simulink model "planar_vtol_sim_HW_08"  (R2018a)
settings: Solver=ode45  StartTime=0.0  StopTime=100  MaxStep=1  MinStep=0.005  RelTol=1e-3
InitFcn:
  | planar_vtol_param
undefined symbols (not defined in the file or in its folder): Pa, planar_vtol_animation, planar_vtol_ctrl
settings Model: Creator=canla  LastModifiedBy=canla
settings OptimizationCC: LifeSpan=inf

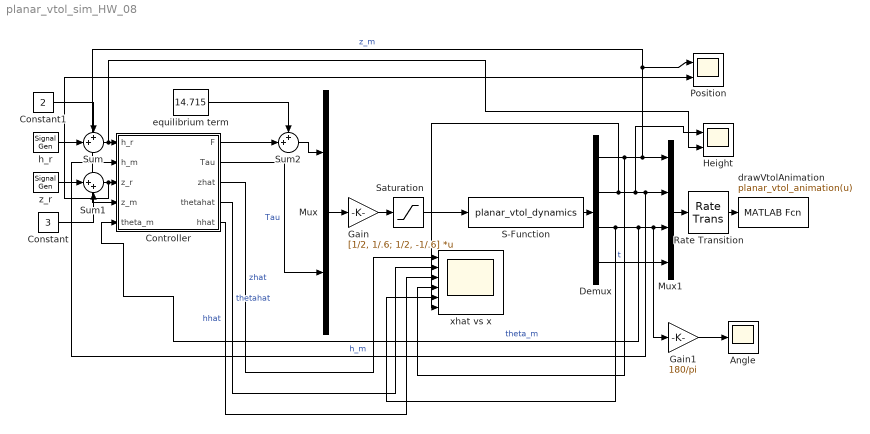
== system planar_vtol_sim_HW_08 ==
  Angle : Scope
  Constant : Constant  Value=3
  Constant1 : Constant  Value=2
  Controller : Subsystem
  Demux : Demux
  Gain : Gain  Gain=[1/2, 1/.6; 1/2, -1/.6]  Multiplication=Matrix(K*u)
  Gain1 : Gain  Gain=180/pi
  Height : Scope  NumInputPorts=2
  Mux : Mux  Inputs=2
  Mux1 : Mux
  Position : Scope  NumInputPorts=2
  Rate Transition : RateTransition  OutPortSampleTime=Pa.t_plot
  S-Function : S-Function  FunctionName=planar_vtol_dynamics  Parameters=Pa  SFunctionDeploymentMode=off  EnableBusSupport=off
  Saturation : Saturate  UpperLimit=Pa.F_max  LowerLimit=-Pa.F_max
  Sum : Sum  Inputs=++|
  Sum1 : Sum  Inputs=|++
  Sum2 : Sum  Inputs=++|
  drawVtolAnimation : MATLABFcn  MATLABFcn=planar_vtol_animation(u)  OutputDimensions=0
  equilibrium term : Constant  Value=14.715
  h_r : SignalGenerator  WaveForm=square  Amplitude=0.15  Frequency=0.03
  xhat vs x : Scope  NumInputPorts=6
  z_r : SignalGenerator  WaveForm=square  Amplitude=0.15  Frequency=0.03
  wires:
  Mux/1 -> Gain/1
  S-Function/1 -> Demux/1
  Demux/1 -> xhat vs x/4, Position/1, Controller/4(z_m), Mux1/1  "z_m"
  Demux/2 -> xhat vs x/6, Height/1, Controller/2(h_m), Mux1/2  "h_m"
  Demux/3 -> xhat vs x/5, Controller/5(theta_m), Gain1/1, Mux1/3  "theta_m"
  Demux/4 -> Mux1/4  "t"
  Mux1/1 -> Rate Transition/1
  Rate Transition/1 -> drawVtolAnimation/1
  Gain/1 -> Saturation/1
  Sum/1 -> Height/2, Controller/1(h_r)
  Sum1/1 -> Position/2, Controller/3(z_r)
  h_r/1 -> Sum/2
  z_r/1 -> Sum1/1
  Constant/1 -> Sum1/2
  Constant1/1 -> Sum/1
  Gain1/1 -> Angle/1
  Sum2/1 -> Mux/1
  Saturation/1 -> S-Function/1
  equilibrium term/1 -> Sum2/1
  Controller/1(F) -> Sum2/2
  Controller/3(zhat) -> xhat vs x/1  "zhat"
  Controller/4(thetahat) -> xhat vs x/2  "thetahat"
  Controller/5(hhat) -> xhat vs x/3  "hhat"
  Controller/2(Tau) -> Mux/2  "Tau"

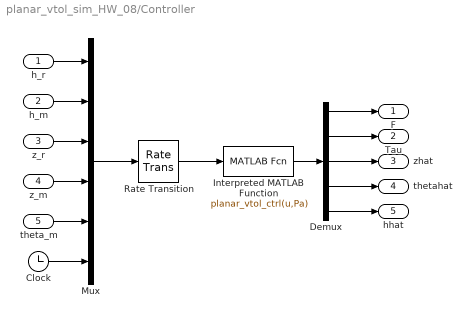
== system planar_vtol_sim_HW_08/Controller ==
  h_r : Inport
  h_m : Inport  Port=2
  z_r : Inport  Port=3
  z_m : Inport  Port=4
  theta_m : Inport  Port=5
  Clock : Clock
  Demux : Demux  Outputs=5
  Interpreted MATLAB Function : MATLABFcn  MATLABFcn=planar_vtol_ctrl(u,Pa)
  Mux : Mux  Inputs=6
  Rate Transition : RateTransition  OutPortSampleTime=Pa.Ts
  F : Outport
  Tau : Outport  Port=2
  zhat : Outport  Port=3
  thetahat : Outport  Port=4
  hhat : Outport  Port=5
  wires:
  h_r/1 -> Mux/1
  h_m/1 -> Mux/2
  z_r/1 -> Mux/3
  z_m/1 -> Mux/4
  theta_m/1 -> Mux/5
  Clock/1 -> Mux/6
  Mux/1 -> Rate Transition/1
  Rate Transition/1 -> Interpreted MATLAB Function/1
  Interpreted MATLAB Function/1 -> Demux/1
  Demux/1 -> F/1
  Demux/2 -> Tau/1
  Demux/3 -> zhat/1
  Demux/4 -> thetahat/1
  Demux/5 -> hhat/1
